simulink model "eclib"  (Simulink 7.8)
settings: Solver=ode45  StartTime=0.0  StopTime=10.0  RelTol=1e-3
settings Model: Creator=root  LastModifiedBy=root  ExtModeAutoUpdateStatusClock=off
settings OptimizationCC: InitFltsAndDblsToZero=on
settings DebuggingCC: SaveWithParameterizedLinksMsg=none  SignalResolutionControl=TryResolveAllWithWarning  MultiTaskDSMMsg=warning  MultiTaskCondExecSysMsg=none  FcnCallInpInsideContextMsg=Use local settings  StrictBusMsg=None
settings RTWCC: IncludeERTFirstTime=on
settings GRTTargetCC: TargetFcnLib=ansi_tfl_tmw.mat

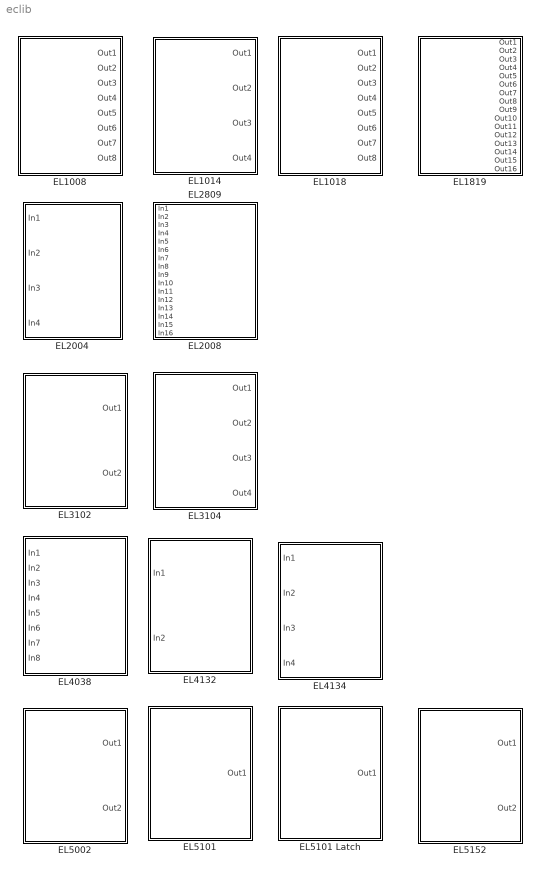
== system eclib ==
  EL1008 : Subsystem  mask(EL1008){link_id=0}
      mask prompts: link_id "Link id (>=0)"
  EL1014 : Subsystem  mask(EL1014){link_id=0}
      mask prompts: link_id "Link id (>=0)"
  EL1018 : Subsystem  mask(EL1008){link_id=0}
      mask prompts: link_id "Link id (>=0)"
  EL1819 : Subsystem  mask(EL1819){link_id=0}
      mask prompts: link_id "Link id (>=0)"
  EL2004 : Subsystem  mask(EL2004){link_id=0}
      mask prompts: link_id "Link id (>=0)"
  EL2008 : Subsystem  mask(EL2008){link_id=0}
      mask prompts: link_id "Link id (>=0)"
  EL2809 : Subsystem  mask(EL2809){link_id=1}
      mask prompts: link_id "Link id (>=0)"
  EL3102 : Subsystem  mask(EL3102){link_id=0}
      mask prompts: link_id "Link id (>=0)"
  EL3104 : Subsystem  mask(EL3102){link_id=0}
      mask prompts: link_id "Link id (>=0)"
  EL4038 : Subsystem  mask(EL4038){link_id=0}
      mask prompts: link_id "Link id (>=0)"
  EL4132 : Subsystem  mask(EL4132){link_id=0}
      mask prompts: link_id "Link id (>=0)"
  EL4134 : Subsystem  mask(EL4134){link_id=0}
      mask prompts: link_id "Link id (>=0)"
  EL5002 : Subsystem  mask(EL5101){link_id=0}
      mask prompts: link_id "Link id (>=0)"
  EL5101 : Subsystem  mask(EL5101){link_id=0}
      mask prompts: link_id "Link id (>=0)"
  EL5101 Latch : Subsystem  mask(EL5101){link_id=0}
      mask prompts: link_id "Link id (>=0)"
  EL5152 : Subsystem  mask(EL5102){link_id=0}
      mask prompts: link_id "Link id (>=0)"

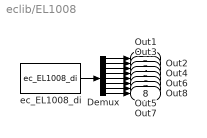
== system eclib/EL1008 ==
  Demux : Demux  Outputs=8
  ec_EL1008_di : S-Function  FunctionName=ec_EL1008_di  Parameters=link_id  EnableBusSupport=off  mask{link_id=link_id}
      mask prompts: link_id "digital in id (start from 1)"
  Out1 : Outport
  Out2 : Outport  Port=2
  Out3 : Outport  Port=3
  Out4 : Outport  Port=4
  Out5 : Outport  Port=5
  Out6 : Outport  Port=6
  Out7 : Outport  Port=7
  Out8 : Outport  Port=8
  wires:
  ec_EL1008_di/1 -> Demux/1
  Demux/1 -> Out1/1
  Demux/2 -> Out2/1
  Demux/3 -> Out3/1
  Demux/4 -> Out4/1
  Demux/5 -> Out5/1
  Demux/6 -> Out6/1
  Demux/7 -> Out7/1
  Demux/8 -> Out8/1

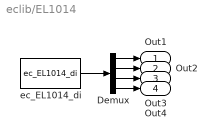
== system eclib/EL1014 ==
  Demux : Demux
  ec_EL1014_di : S-Function  FunctionName=ec_EL1014_di  Parameters=link_id  EnableBusSupport=off  mask{link_id=link_id}
      mask prompts: link_id "digital in id (start from 1)"
  Out1 : Outport
  Out2 : Outport  Port=2
  Out3 : Outport  Port=3
  Out4 : Outport  Port=4
  wires:
  ec_EL1014_di/1 -> Demux/1
  Demux/1 -> Out1/1
  Demux/2 -> Out2/1
  Demux/3 -> Out3/1
  Demux/4 -> Out4/1

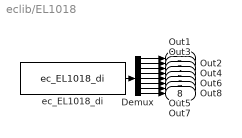
== system eclib/EL1018 ==
  Demux : Demux  Outputs=8
  ec_EL1018_di : S-Function  FunctionName=ec_EL1018_di  Parameters=link_id  EnableBusSupport=off  mask{link_id=link_id}
      mask prompts: link_id "digital in id (start from 1)"
  Out1 : Outport
  Out2 : Outport  Port=2
  Out3 : Outport  Port=3
  Out4 : Outport  Port=4
  Out5 : Outport  Port=5
  Out6 : Outport  Port=6
  Out7 : Outport  Port=7
  Out8 : Outport  Port=8
  wires:
  Demux/8 -> Out8/1
  Demux/7 -> Out7/1
  Demux/6 -> Out6/1
  Demux/5 -> Out5/1
  Demux/4 -> Out4/1
  Demux/3 -> Out3/1
  Demux/2 -> Out2/1
  Demux/1 -> Out1/1
  ec_EL1018_di/1 -> Demux/1

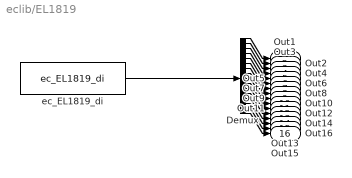
== system eclib/EL1819 ==
  Demux : Demux  Outputs=16
  ec_EL1819_di : S-Function  FunctionName=ec_EL1819_di  Parameters=link_id  EnableBusSupport=off  mask{link_id=link_id}
      mask prompts: link_id "digital in id (start from 1)"
  Out1 : Outport
  Out2 : Outport  Port=2
  Out3 : Outport  Port=3
  Out4 : Outport  Port=4
  Out5 : Outport  Port=5
  Out6 : Outport  Port=6
  Out7 : Outport  Port=7
  Out8 : Outport  Port=8
  Out9 : Outport  Port=9
  Out10 : Outport  Port=10
  Out11 : Outport  Port=11
  Out12 : Outport  Port=12
  Out13 : Outport  Port=13
  Out14 : Outport  Port=14
  Out15 : Outport  Port=15
  Out16 : Outport  Port=16
  wires:
  Demux/16 -> Out16/1
  Demux/15 -> Out15/1
  Demux/14 -> Out14/1
  Demux/13 -> Out13/1
  Demux/12 -> Out12/1
  Demux/11 -> Out11/1
  Demux/10 -> Out10/1
  Demux/9 -> Out9/1
  Demux/8 -> Out8/1
  Demux/7 -> Out7/1
  Demux/6 -> Out6/1
  Demux/5 -> Out5/1
  Demux/4 -> Out4/1
  Demux/3 -> Out3/1
  Demux/2 -> Out2/1
  Demux/1 -> Out1/1
  ec_EL1819_di/1 -> Demux/1

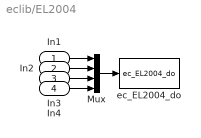
== system eclib/EL2004 ==
  In1 : Inport
  In2 : Inport  Port=2
  In3 : Inport  Port=3
  In4 : Inport  Port=4
  Mux : Mux
  ec_EL2004_do : S-Function  FunctionName=ec_EL2004_do  Parameters=link_id  EnableBusSupport=off  mask{link_id=link_id}
      mask prompts: link_id "digital out id (start from 1)"
  wires:
  Mux/1 -> ec_EL2004_do/1
  In1/1 -> Mux/1
  In2/1 -> Mux/2
  In3/1 -> Mux/3
  In4/1 -> Mux/4

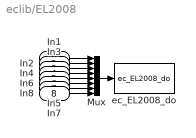
== system eclib/EL2008 ==
  In1 : Inport
  In2 : Inport  Port=2
  In3 : Inport  Port=3
  In4 : Inport  Port=4
  In5 : Inport  Port=5
  In6 : Inport  Port=6
  In7 : Inport  Port=7
  In8 : Inport  Port=8
  Mux : Mux  Inputs=8
  ec_EL2008_do : S-Function  FunctionName=ec_EL2008_do  Parameters=link_id  EnableBusSupport=off  mask{link_id=link_id}
      mask prompts: link_id "digital out id (start from 1)"
  wires:
  Mux/1 -> ec_EL2008_do/1
  In1/1 -> Mux/1
  In2/1 -> Mux/2
  In3/1 -> Mux/3
  In4/1 -> Mux/4
  In5/1 -> Mux/5
  In6/1 -> Mux/6
  In7/1 -> Mux/7
  In8/1 -> Mux/8

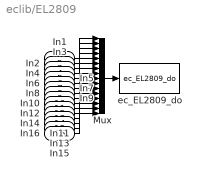
== system eclib/EL2809 ==
  In1 : Inport
  In2 : Inport  Port=2
  In3 : Inport  Port=3
  In4 : Inport  Port=4
  In5 : Inport  Port=5
  In6 : Inport  Port=6
  In7 : Inport  Port=7
  In8 : Inport  Port=8
  In9 : Inport  Port=9
  In10 : Inport  Port=10
  In11 : Inport  Port=11
  In12 : Inport  Port=12
  In13 : Inport  Port=13
  In14 : Inport  Port=14
  In15 : Inport  Port=15
  In16 : Inport  Port=16
  Mux : Mux  Inputs=16
  ec_EL2809_do : S-Function  FunctionName=ec_EL2809_do  Parameters=link_id  EnableBusSupport=off  mask{link_id=link_id}
      mask prompts: link_id "digital out id (start from 1)"
  wires:
  Mux/1 -> ec_EL2809_do/1
  In1/1 -> Mux/1
  In2/1 -> Mux/2
  In3/1 -> Mux/3
  In4/1 -> Mux/4
  In5/1 -> Mux/5
  In6/1 -> Mux/6
  In7/1 -> Mux/7
  In8/1 -> Mux/8
  In9/1 -> Mux/9
  In10/1 -> Mux/10
  In11/1 -> Mux/11
  In12/1 -> Mux/12
  In13/1 -> Mux/13
  In14/1 -> Mux/14
  In15/1 -> Mux/15
  In16/1 -> Mux/16

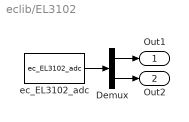
== system eclib/EL3102 ==
  Demux : Demux  Outputs=2
  ec_EL3102_adc : S-Function  FunctionName=ec_EL3102_adc  Parameters=link_id  EnableBusSupport=off  mask{link_id=link_id}
      mask prompts: link_id "analog in id (start from 1)"
  Out1 : Outport
  Out2 : Outport  Port=2
  wires:
  ec_EL3102_adc/1 -> Demux/1
  Demux/1 -> Out1/1
  Demux/2 -> Out2/1

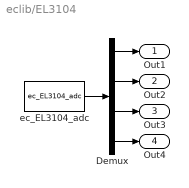
== system eclib/EL3104 ==
  Demux : Demux
  ec_EL3104_adc : S-Function  FunctionName=ec_EL3104_adc  Parameters=link_id  EnableBusSupport=off  mask{link_id=link_id}
      mask prompts: link_id "analog in id (start from 1)"
  Out1 : Outport
  Out2 : Outport  Port=2
  Out3 : Outport  Port=3
  Out4 : Outport  Port=4
  wires:
  ec_EL3104_adc/1 -> Demux/1
  Demux/1 -> Out1/1
  Demux/2 -> Out2/1
  Demux/3 -> Out3/1
  Demux/4 -> Out4/1

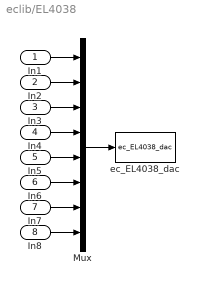
== system eclib/EL4038 ==
  In1 : Inport
  In2 : Inport  Port=2
  In3 : Inport  Port=3
  In4 : Inport  Port=4
  In5 : Inport  Port=5
  In6 : Inport  Port=6
  In7 : Inport  Port=7
  In8 : Inport  Port=8
  Mux : Mux  Inputs=8
  ec_EL4038_dac : S-Function  FunctionName=ec_EL4038_dac  Parameters=link_id  EnableBusSupport=off  mask{link_id=link_id}
      mask prompts: link_id "analog out id (start from 1)"
  wires:
  Mux/1 -> ec_EL4038_dac/1
  In1/1 -> Mux/1
  In2/1 -> Mux/2
  In8/1 -> Mux/8
  In7/1 -> Mux/7
  In6/1 -> Mux/6
  In5/1 -> Mux/5
  In4/1 -> Mux/4
  In3/1 -> Mux/3

== system eclib/EL4132 ==
  In1 : Inport
  In2 : Inport  Port=2
  Mux : Mux  Inputs=2
  ec_EL4132_dac : S-Function  FunctionName=ec_EL4132_dac  Parameters=link_id  EnableBusSupport=off  mask{link_id=link_id}
      mask prompts: link_id "analog out id (start from 1)"
  wires:
  Mux/1 -> ec_EL4132_dac/1
  In1/1 -> Mux/1
  In2/1 -> Mux/2

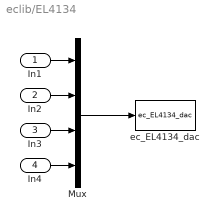
== system eclib/EL4134 ==
  In1 : Inport
  In2 : Inport  Port=2
  In3 : Inport  Port=3
  In4 : Inport  Port=4
  Mux : Mux
  ec_EL4134_dac : S-Function  FunctionName=ec_EL4134_dac  Parameters=link_id  EnableBusSupport=off  mask{link_id=link_id}
      mask prompts: link_id "analog out id (start from 1)"
  wires:
  Mux/1 -> ec_EL4134_dac/1
  In1/1 -> Mux/1
  In2/1 -> Mux/2
  In3/1 -> Mux/3
  In4/1 -> Mux/4

== system eclib/EL5002 ==
  Demux : Demux  Outputs=2
  ec_EL5101_enc : S-Function  FunctionName=ec_EL5002_ssi  Parameters=link_id  EnableBusSupport=off  mask{link_id=link_id}
      mask prompts: link_id "encoder in id (start from 1)"
  Out1 : Outport
  Out2 : Outport  Port=2
  wires:
  ec_EL5101_enc/1 -> Demux/1
  Demux/1 -> Out1/1
  Demux/2 -> Out2/1

== system eclib/EL5101 ==
  ec_EL5101_enc : S-Function  FunctionName=ec_EL5101_enc  Parameters=link_id  EnableBusSupport=off  mask{link_id=link_id}
      mask prompts: link_id "encoder in id (start from 1)"
  Out1 : Outport
  wires:
  ec_EL5101_enc/1 -> Out1/1

== system eclib/EL5101 Latch ==
  ec_EL5101_enc : S-Function  FunctionName=ec_EL5101_latch  Parameters=link_id  EnableBusSupport=off  mask{link_id=link_id}
      mask prompts: link_id "encoder in id (start from 1)"
  Out1 : Outport
  wires:
  ec_EL5101_enc/1 -> Out1/1

== system eclib/EL5152 ==
  Demux : Demux  Outputs=2
  ec_EL5102_enc : S-Function  FunctionName=ec_EL5152_enc  Parameters=link_id  EnableBusSupport=off  mask{link_id=link_id}
      mask prompts: link_id "encoder in id (start from 1)"
  Out1 : Outport
  Out2 : Outport  Port=2
  wires:
  ec_EL5102_enc/1 -> Demux/1
  Demux/1 -> Out1/1
  Demux/2 -> Out2/1
